simulink model "MalhaFechadaTorradeira"  (R2020b)
settings: Solver=VariableStepAuto  StartTime=0.0  StopTime=4  MaxStep=1e-3  RelTol=1e-3
libraries: Library_Aula01 x2, simulink x1
settings Model: Creator=carlo  LastModifiedBy=carlo
settings DataIOCC: ReturnWorkspaceOutputs=off
settings DebuggingCC: PregeneratedLibrarySubsystemCodeDiagnostic=none  ArithmeticOperatorsInVariantConditions=warning
settings SFSimCC: SimUseLocalCustomCode=off  CustomCodeUndefinedFunction=UseInterfaceOnly
settings RTWCC: RTWUseLocalCustomCode=off

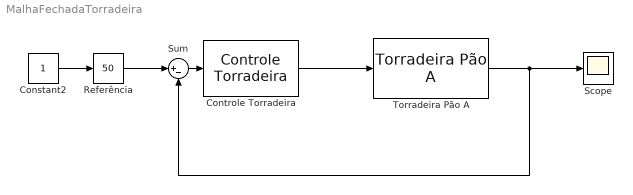
== system MalhaFechadaTorradeira ==
  Constant2 : Constant
  Controle Torradeira : Library_Aula01/Controle Torradeira  SystemSampleTime=-1  VariantActivationTime=update diagram  Latency=0  AutoFrameSizeCalculation=off
  Referência : simulink/Math Operations/Slider Gain  gain=50  low=0  high=100
  Scope : Scope
  Sum : Sum  Inputs=|+-
  Torradeira Pão A : Library_Aula01/Torradeira Pão A  SystemSampleTime=-1  VariantActivationTime=update diagram  Latency=0  AutoFrameSizeCalculation=off
  wires:
  Referência/1 -> Sum/1
  Constant2/1 -> Referência/1
  Sum/1 -> Controle Torradeira/1
  Torradeira Pão A/1 -> Sum/2, Scope/1
  Controle Torradeira/1 -> Torradeira Pão A/1
